simulink model "aircraft_model"  (R2026a)
settings: Solver=VariableStepAuto
settings Model: Creator=Shreyan Dey  LastModifiedBy=Shreyan Dey

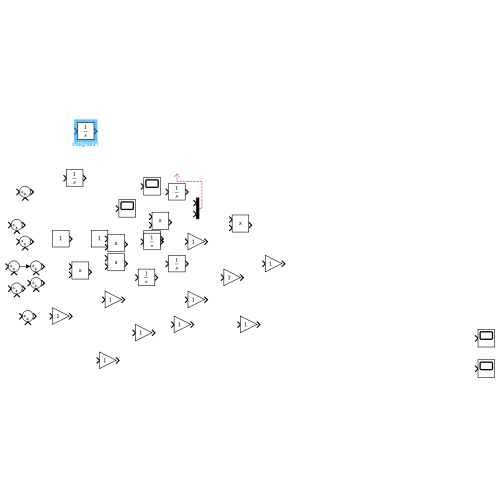
[thumbnail: Simulink's stored preview of the top-level diagram]
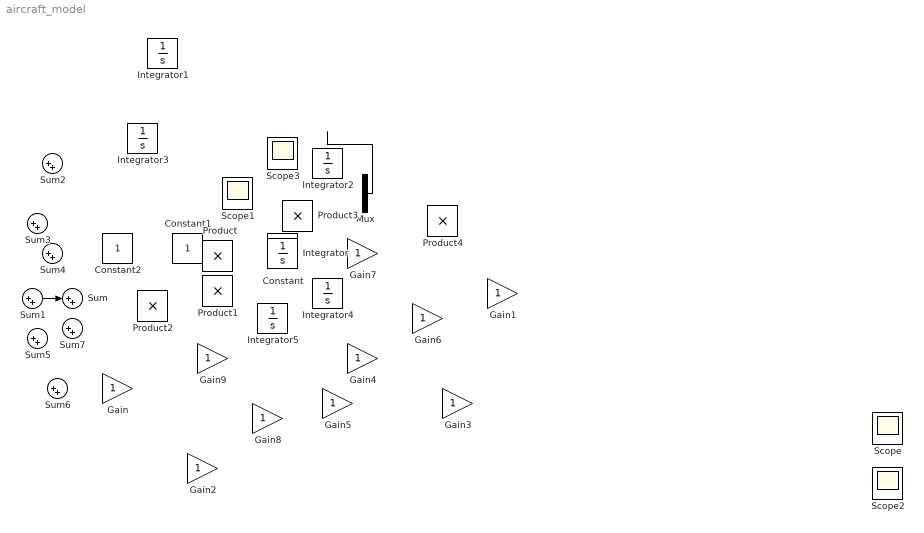
== system aircraft_model ==
  Constant : Constant
  Constant1 : Constant
  Constant2 : Constant
  Gain{,1..9} (10 alike) : Gain
  Integrator{,2..5} (5 alike) : Integrator
  Integrator1 : Integrator  ContinuousStateAttributes=Throttle
  Mux : Mux  Inputs=2
  Product{,1..4} (5 alike) : Product
  Scope{,1..3} (4 alike) : Scope
      Scope2 settings: DataLoggingVariableName=ScopeData2
      Scope3 settings: DataLoggingVariableName=ScopeData3
  Sum{,1..7} (8 alike) : Sum  Inputs=|++
  wires:
  Mux/1 -> ?
  Sum1/1 -> Sum/1
